simulink model "LAB1_interface"  (R2023b)
settings: Solver=FixedStepAuto  StartTime=0.0  StopTime=54  FixedStep=0.01  RelTol=1e-3
values from neighbouring files (symbols this model uses):
  motor_B = 0.0001    [example_data_LAB1.mat]    (also in motor_params.m)
  motor_J = 0.001    [example_data_LAB1.mat]    (also in motor_params.m)
  motor_K = 0.05    [example_data_LAB1.mat]    (also in motor_params.m)
  motor_L = 0.016    [example_data_LAB1.mat]    (also in motor_params.m)
  motor_R = 22    [example_data_LAB1.mat]    (also in motor_params.m)
undefined symbols (not defined in the file or in its folder): LF
libraries: simulink x4, instrumentseriallib x4, hdlsllib x1
settings Model: Creator=tanawatp  LastModifiedBy=tanawatp

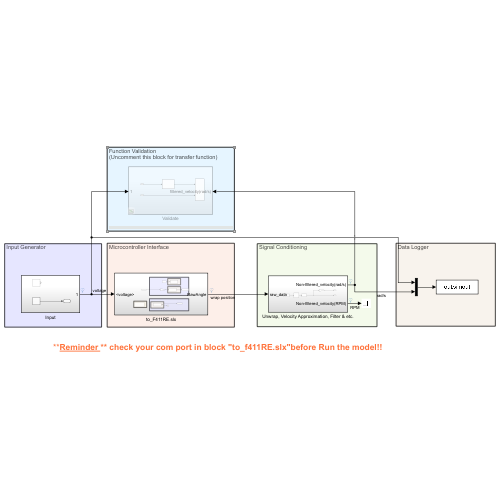
[thumbnail: Simulink's stored preview of the top-level diagram]
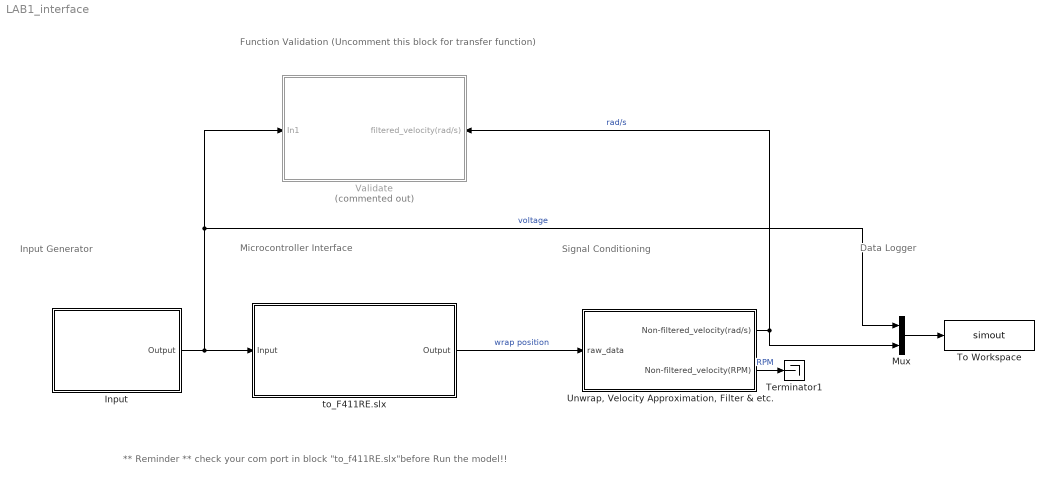
== system LAB1_interface ==
  note: ** Reminder ** check your com port in block "to_f411RE.slx"before Run the model!!
  note: Signal Conditioning
  note: Function Validation
      | (Uncomment this block for transfer function)
  note: Input Generator
  note: Data Logger
  note: Microcontroller Interface
  Input : Subsystem
  Mux : Mux  Inputs=2
  Terminator1 : Terminator
  To Workspace : ToWorkspace  VariableName=simout  SaveFormat=Timeseries  SampleTime=-1
  "Unwrap, Velocity Approximation, Filter & etc." : Subsystem
  Validate : Subsystem  Commented=on
      settings: PortSchema="{\"entries\":[{\"content\":{\"sides\":[{\"content\":{\"connectorIds\":[\"In1\"]},\"type\":\"ConnectorPlacement.EquallySpacedRectSide\",\"uuid\":\"2e198c62-3f63-40d2-bae8-9fd8fef67e0c\"},{\"content\":{\"connectorIds\":[\"In2\"],\"side\":\"RIGHT\"},\"type\":\"ConnectorPlacement.EquallySpacedRectSide\",\"uuid\":\"8587534e-14f7-4890-8a03-94178e65376b\"},{\"content\":{\"side\":\"TOP\"},\"type\":\"ConnectorPlacement.EquallySpacedRectSide\",\"uuid\":\"1b7cad7c-cb5d-42c2-b7c5-a9278b867159\"}]},\"type\":\"ConnectorPlacement.EquallySpacedConnector\",\"uuid\":\"07c3edf9-7db3-4a0b-af16-87d57ef9c94a\"}],\"packageUris\":[\"http://schema.mathworks.com/mf0/Connector/R2020b\"],\"version\":\"1.0\"}"
  to_F411RE.slx : Subsystem
  wires:
  Mux/1 -> To Workspace/1
  Input/1(Output) -> Validate/1(In1), Mux/1, to_F411RE.slx/1(Input)  "voltage"
  to_F411RE.slx/1(Output) -> "Unwrap, Velocity Approximation, Filter & etc."/1(raw_data)  "wrap position"
  "Unwrap, Velocity Approximation, Filter & etc."/1(Non-filtered_velocity(rad/s)) -> Mux/2, Validate/2(filtered_velocity(rad/s))  "rad/s"
  "Unwrap, Velocity Approximation, Filter & etc."/2(Non-filtered_velocity(RPM)) -> Terminator1/1  "RPM"

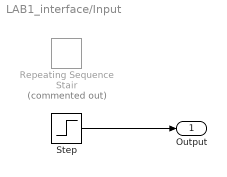
== system LAB1_interface/Input ==
  Repeating Sequence Stair : simulink/Sources/Repeating Sequence Stair  Commented=on  OutValues=[0 5 0 6 0 7 0 8 0 9 0 10 0 11 0 12 0 0]  tsamp=3  OutMin=[]  OutMax=[]  OutDataTypeStr=double  OutputDataTypeScalingMode=double  OutDataType=fixdt(0,8)  ConRadixGroup=Best Precision: Vector-wise  OutScaling=2^-12
  Step : Step  SampleTime=0
  Output : Outport
  wires:
  Step/1 -> Output/1

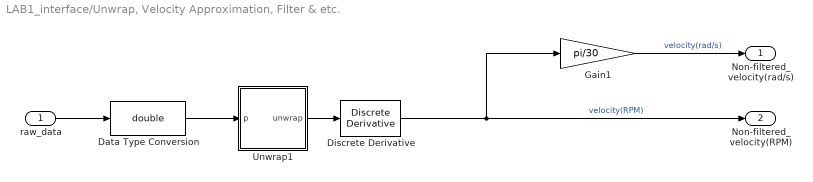
== system LAB1_interface/Unwrap, Velocity Approximation, Filter & etc. ==
  raw_data : Inport
  Data Type Conversion : DataTypeConversion  OutDataTypeStr=double  SaturateOnIntegerOverflow=off  RndMeth=Floor
  Discrete Derivative : simulink/Discrete/Discrete Derivative  gainval=60 / 4095  ICPrevScaledInput=0.0  OutMin=[]  OutMax=[]  OutDataType=fixdt(1, 16)  OutScaling=2^-10  DoSatur=off
  Gain1 : Gain  Gain=pi/30
  Unwrap1 : Subsystem
  Non-filtered_velocity(rad/s) : Outport
  Non-filtered_velocity(RPM) : Outport  Port=2
  wires:
  Unwrap1/1(unwrap) -> Discrete Derivative/1
  raw_data/1 -> Data Type Conversion/1
  Discrete Derivative/1 -> Non-filtered_velocity(RPM)/1, Gain1/1  "velocity(RPM)"
  Data Type Conversion/1 -> Unwrap1/1(p)
  Gain1/1 -> Non-filtered_velocity(rad/s)/1  "velocity(rad/s)"

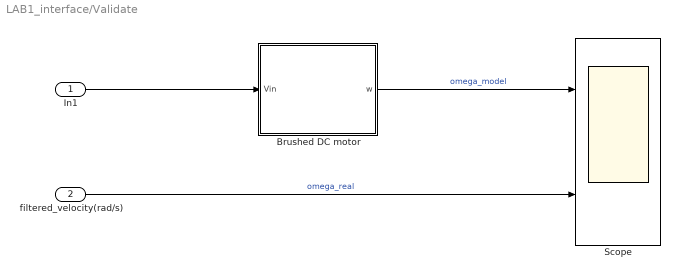
== system LAB1_interface/Validate ==
  In1 : Inport
  filtered_velocity(rad/s) : Inport  Port=2
  Brushed DC motor : Subsystem
  Scope : Scope  NumInputPorts=2
  wires:
  filtered_velocity(rad/s)/1 -> Scope/2  "omega_real"
  In1/1 -> Brushed DC motor/1(Vin)
  Brushed DC motor/1(w) -> Scope/1  "omega_model"

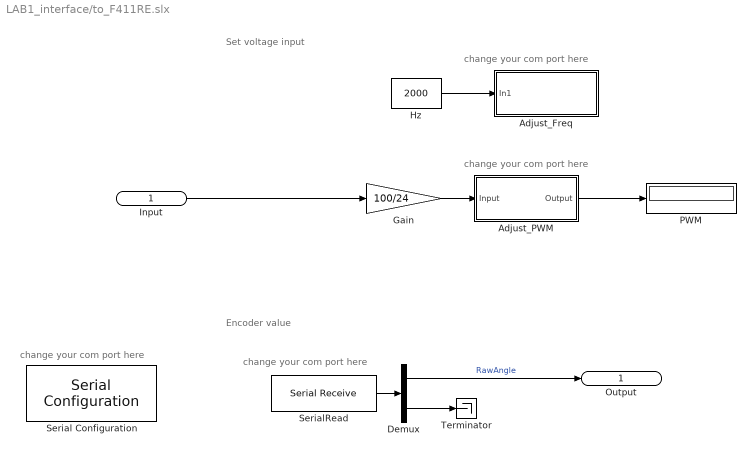
== system LAB1_interface/to_F411RE.slx ==
  note: change your com port here
  note: Encoder value
  note: Set voltage input
  note: change your com port here
  note: change your com port here
  note: change your com port here
  Input : Inport
  Adjust_Freq : Subsystem
  Adjust_PWM : Subsystem
  Demux : Demux  Outputs=2
  Gain : Gain  Gain=100/24  OutDataTypeStr=int8
  Hz : Constant  Value=2000  OutDataTypeStr=double
  PWM : Display
  Serial Configuration : instrumentseriallib/Serial Configuration  Priority=-200000  PortSel=COM6  Port=COM6  ComPort=COM6  BaudRate=115200  DataBits=8  Parity=none  StopBits=1  ByteOrder=little-endian  FlowControl=none  Timeout=10  SimulateUsing=Interpreted execution  BlockInModel=on  aMode=1
  SerialRead : instrumentseriallib/Serial Receive  Priority=1  PortSel=COM6  Port=COM6  ComPort=COM6  DataType=uint16  SaveDataType=uint8  ToggleHeader=on  Header=[69]  ToggleTerminator=on  Terminator=LF ('\n')  CustomTerminator=[]  InputFormat=Column major  ToggleDataSize=on  DataSize=[2]  EnableBlockingMode=on  ActionDataUnavailable=Output last received value  ActionWhenDataUnavailable=Output last received value  CustomValue=0  SampleTime=-1  SimulateUsing=Interpreted execution  BlockInModel=on  aMode=1
  Terminator : Terminator
  Output : Outport
  wires:
  Demux/1 -> Output/1  "RawAngle"
  Gain/1 -> Adjust_PWM/1(Input)
  Input/1 -> Gain/1
  Hz/1 -> Adjust_Freq/1(In1)
  Adjust_PWM/1(Output) -> PWM/1
  SerialRead/1 -> Demux/1
  Demux/2 -> Terminator/1

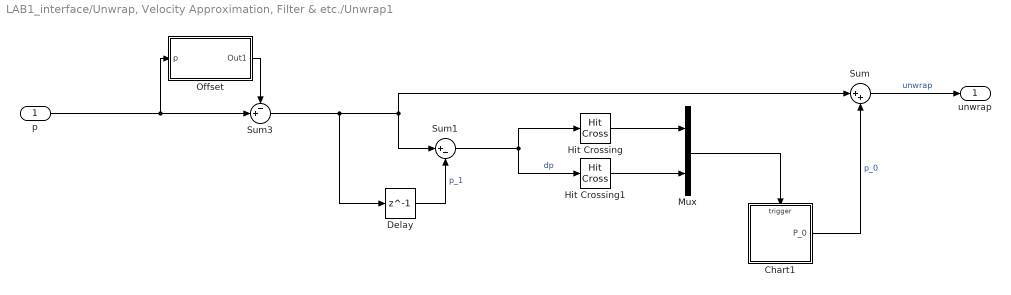
== system LAB1_interface/Unwrap, Velocity Approximation, Filter & etc./Unwrap1 ==
  p : Inport
  Chart1 : Stateflow chart  TreatAsAtomicUnit=on
  Delay : Delay  DelayLength=1
  Hit Crossing : HitCross  HitCrossingOffset=0.7*65535  HitCrossingDirection=rising
  Hit Crossing1 : HitCross  HitCrossingOffset=-0.7*65535  HitCrossingDirection=falling
  Mux : Mux  Inputs=2
  Offset : Subsystem
  Sum : Sum  Inputs=|++
  Sum1 : Sum  Inputs=|+-
  Sum3 : Sum  Inputs=-+|
  unwrap : Outport
  wires:
  Hit Crossing/1 -> Mux/1
  Hit Crossing1/1 -> Mux/2
  Chart1/1(P_0) -> Sum/2  "p_0"
  Sum1/1 -> Hit Crossing1/1, Hit Crossing/1  "dp"
  Sum3/1 -> Delay/1, Sum/1, Sum1/1
  Mux/1 -> Chart1/Trigger
  Sum/1 -> unwrap/1  "unwrap"
  Delay/1 -> Sum1/2  "p_1"
  Offset/1(Out1) -> Sum3/1
  p/1 -> Sum3/2, Offset/1(p)

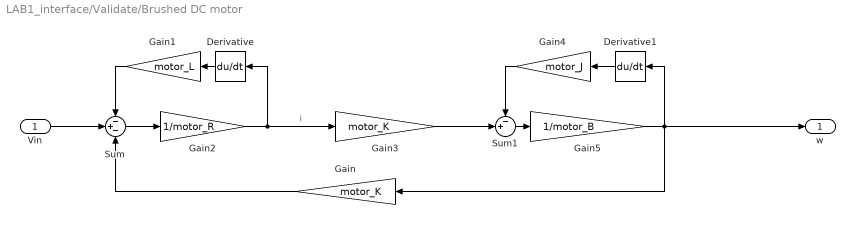
== system LAB1_interface/Validate/Brushed DC motor ==
  Vin : Inport
  Derivative : Derivative
  Derivative1 : Derivative
  Gain : Gain  Gain=motor_K
  Gain1 : Gain  Gain=motor_L
  Gain2 : Gain  Gain=1/motor_R
  Gain3 : Gain  Gain=motor_K
  Gain4 : Gain  Gain=motor_J
  Gain5 : Gain  Gain=1/motor_B
  Sum : Sum  Inputs=-+-
  Sum1 : Sum  Inputs=-+|
  w : Outport
  wires:
  Derivative/1 -> Gain1/1
  Gain5/1 -> w/1, Gain/1, Derivative1/1
  Gain1/1 -> Sum/1
  Gain4/1 -> Sum1/1
  Sum/1 -> Gain2/1
  Gain3/1 -> Sum1/2
  Sum1/1 -> Gain5/1
  Gain/1 -> Sum/3
  Derivative1/1 -> Gain4/1
  Gain2/1 -> Derivative/1, Gain3/1  "i"
  Vin/1 -> Sum/2

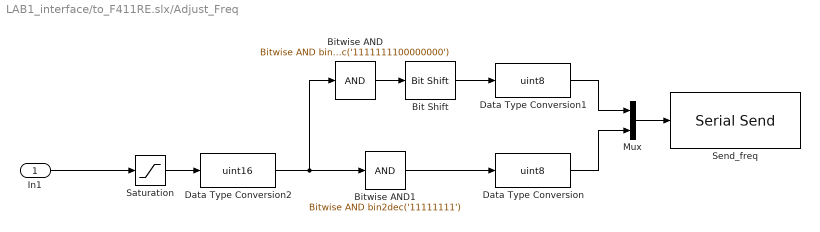
== system LAB1_interface/to_F411RE.slx/Adjust_Freq ==
  In1 : Inport
  Bit Shift : hdlsllib/Logic and Bit Operations/Bit Shift  mode=Shift Right Logical  N=8
  Bitwise AND : simulink/Logic and Bit Operations/Bitwise Operator  logicop=AND  UseBitMask=on  BitMask=bin2dec('1111111100000000')  BitMaskRealWorld=Stored Integer
  Bitwise AND1 : simulink/Logic and Bit Operations/Bitwise Operator  logicop=AND  UseBitMask=on  BitMask=bin2dec('11111111')  BitMaskRealWorld=Stored Integer
  Data Type Conversion : DataTypeConversion  OutDataTypeStr=uint8  SaturateOnIntegerOverflow=off  RndMeth=Floor
  Data Type Conversion1 : DataTypeConversion  OutDataTypeStr=uint8  SaturateOnIntegerOverflow=off  RndMeth=Floor
  Data Type Conversion2 : DataTypeConversion  OutDataTypeStr=uint16  SaturateOnIntegerOverflow=off  RndMeth=Floor
  Mux : Mux  Inputs=2
  Saturation : Saturate  UpperLimit=20000  LowerLimit=5
  Send_freq : instrumentseriallib/Serial Send  Priority=1  PortSel=COM6  Port=COM6  ComPort=COM6  Header=[69]  Terminator=<none>  CustomTerminator=[123]  EnableBlockingMode=on  SimulateUsing=Interpreted execution  BlockInModel=on  aMode=1
  wires:
  Mux/1 -> Send_freq/1
  Saturation/1 -> Data Type Conversion2/1
  Data Type Conversion/1 -> Mux/2
  Bitwise AND/1 -> Bit Shift/1
  Bitwise AND1/1 -> Data Type Conversion/1
  Data Type Conversion2/1 -> Bitwise AND1/1, Bitwise AND/1
  Data Type Conversion1/1 -> Mux/1
  Bit Shift/1 -> Data Type Conversion1/1
  In1/1 -> Saturation/1

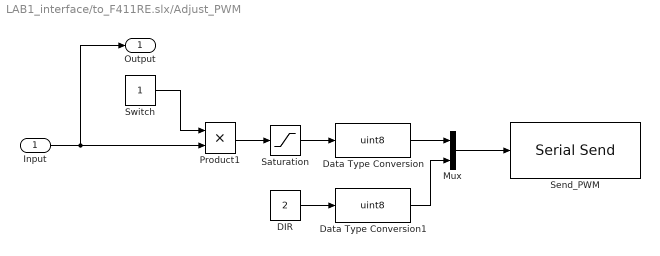
== system LAB1_interface/to_F411RE.slx/Adjust_PWM ==
  Input : Inport
  "DIR " : Constant  Value=2
  Data Type Conversion : DataTypeConversion  OutDataTypeStr=uint8  SaturateOnIntegerOverflow=off  RndMeth=Floor
  Data Type Conversion1 : DataTypeConversion  OutDataTypeStr=uint8  SaturateOnIntegerOverflow=off  RndMeth=Floor
  Mux : Mux  Inputs=2
  Product1 : Product
  Saturation : Saturate  UpperLimit=200  LowerLimit=0
  Send_PWM : instrumentseriallib/Serial Send  Priority=1  PortSel=COM6  Port=COM6  ComPort=COM6  Header=[70]  Terminator=<none>  CustomTerminator=[123]  EnableBlockingMode=on  SimulateUsing=Interpreted execution  BlockInModel=on  aMode=1
  Switch : Constant
  Output : Outport
  wires:
  Input/1 -> Output/1, Product1/2
  Switch/1 -> Product1/1
  Product1/1 -> Saturation/1
  Data Type Conversion/1 -> Mux/1
  Saturation/1 -> Data Type Conversion/1
  "DIR "/1 -> Data Type Conversion1/1
  Mux/1 -> Send_PWM/1
  Data Type Conversion1/1 -> Mux/2

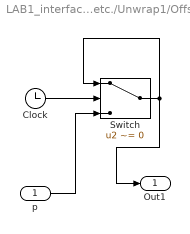
== system LAB1_interface/Unwrap, Velocity Approximation, Filter & etc./Unwrap1/Offset ==
  p : Inport
  Clock : Clock
  Switch : Switch  Criteria=u2 ~= 0  SaturateOnIntegerOverflow=off  InputSameDT=off
  Out1 : Outport
  wires:
  Clock/1 -> Switch/2
  Switch/1 -> Out1/1, Switch/1
  p/1 -> Switch/3

== stateflow chart LAB1_interface/Unwrap, Velocity Approximation, Filter & etc./Unwrap1/Chart1 ==
  settings: executeAtInitialization=1
  state initial
  (default) -> initial : {P_0 = 0;}
  initial -> initial [order 2] : e1{P_0 = P_0-65535;}
  initial -> initial [order 1] : e2{P_0 = P_0+65535;}
  data: P_0 output
  events: e1 input RISING_EDGE_EVENT; e2 input RISING_EDGE_EVENT
